simulink model "sim_mdl"  (R2020b)
settings: Solver=FixedStepAuto  StartTime=0.0  StopTime=stoptime  FixedStep=h  MaxStep=1  RelTol=1e-3  AbsTol=1e-6
values from neighbouring files (symbols this model uses):
  ref_select = 1    [Init_general.m]
  strategy_select = 4    [Init_general.m]
undefined symbols (not defined in the file or in its folder): p
settings Model: PauseTimes=3  PacingRate=0.100000  Creator=nobel  LastModifiedBy=natha

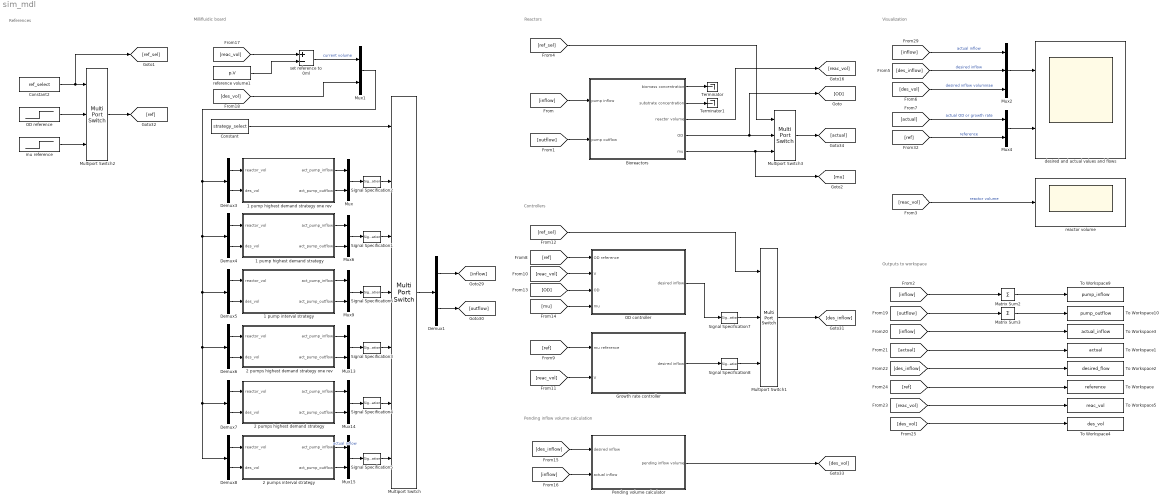
== system sim_mdl ==
  note: Outputs to workspace
  note: Pending inflow volume calculation
  note: Controllers
  note: Millifluidic board
  note: References
  note: Visualization
  note: Reactors
  1 pump highest demand strategy : Stateflow chart  TreatAsAtomicUnit=on  mask{p=p}
      mask prompts: p "Reactor Parameter Struct"
  1 pump highest demand strategy one rev : Stateflow chart  TreatAsAtomicUnit=on  mask{p=p}
      mask prompts: p "Reactor Parameter Struct"
  1 pump interval strategy : Stateflow chart  TreatAsAtomicUnit=on  mask{p=p}
      mask prompts: p "Reactor Parameter Struct"
  2 pumps highest demand strategy : Stateflow chart  TreatAsAtomicUnit=on  mask{p=p}
      mask prompts: p "Reactor Parameter Struct"
  2 pumps highest demand strategy one rev : Stateflow chart  TreatAsAtomicUnit=on  mask{p=p}
      mask prompts: p "Reactor Parameter Struct"
  2 pumps interval strategy : Stateflow chart  TreatAsAtomicUnit=on  mask{p=p}
      mask prompts: p "Reactor Parameter Struct"
  Bioreactors : Subsystem  mask{p=p}
      mask prompts: p "Reactor Parameter Struct"
  Constant : Constant  Value=strategy_select
  Constant2 : Constant  Value=ref_select
  Demux{1,3..8} (7 alike) : Demux  Outputs=2
  Growth rate controller : Subsystem  mask{p=p}
      mask prompts: p "Reactor Parameter Struct"
  Matrix Sum2 : Sum  Inputs=+
  Matrix Sum3 : Sum  Inputs=+
  Multiport Switch : MultiPortSwitch  Inputs=6
  Multiport Switch1 : MultiPortSwitch  Inputs=2
  Multiport Switch2 : MultiPortSwitch  Inputs=2
  Multiport Switch3 : MultiPortSwitch  Inputs=2
  Mux{,1,4,6,9,13..15} (8 alike) : Mux  Inputs=2
  Mux2 : Mux  Inputs=3
  OD controller : Subsystem  mask{p=p}
      mask prompts: p "Reactor Parameter Struct"
  OD reference : Step  Time=p.OD.step_time  Before=p.OD.init_val  After=p.OD.final_val  SampleTime=0  mask{p=p}
      mask prompts: p "Reactor Parameter Struct"
  Pending volume calculator : Subsystem
  Signal Specification{1..6} (6 alike) : SignalSpecification  Dimensions=2*p.num_reac
  Signal Specification7 : SignalSpecification  Dimensions=p.num_reac
  Signal Specification8 : SignalSpecification  Dimensions=p.num_reac
  Terminator : Terminator
  Terminator1 : Terminator
  To Workspace : ToWorkspace  VariableName=reference  SampleTime=-1
  To Workspace1 : ToWorkspace  VariableName=actual  SampleTime=-1
  To Workspace10 : ToWorkspace  VariableName=pump_outflow  SampleTime=-1
      settings: Save2DSignal=2-D array (concatenate along first dimension)
  To Workspace2 : ToWorkspace  VariableName=desired_flow  SampleTime=-1
  To Workspace3 : ToWorkspace  VariableName=actual_inflow  SampleTime=-1
      settings: Save2DSignal=2-D array (concatenate along first dimension)
  To Workspace4 : ToWorkspace  VariableName=des_vol  SampleTime=-1
  To Workspace5 : ToWorkspace  VariableName=reac_vol  SampleTime=-1
  To Workspace9 : ToWorkspace  VariableName=pump_inflow  SampleTime=-1
      settings: Save2DSignal=2-D array (concatenate along first dimension)
  desired and actual values and flows : Scope  NumInputPorts=2
  mu reference : Step  Time=p.growth_rate.step_time  Before=p.growth_rate.init_val  After=p.growth_rate.final_val  SampleTime=0  mask{p=p}
      mask prompts: p "Reactor Parameter Struct"
  reactor volume : Scope
  reference volume1 : Constant  Value=p.V  mask{p=p}
      mask prompts: p "Reactor Parameter Struct"
  set reference to 0ml : Sum  Inputs=+-
  wires:
  Multiport Switch2/1 -> [ref]
  Demux1/2 -> [outflow]
  Demux1/1 -> [inflow]
  [ref] -> Mux4/2  "reference"
  [des_inflow] -> Mux2/2  "desired inflow"
  [des_vol] -> Mux2/3  "desired inflow voluminae"
  Mux4/1 -> desired and actual values and flows/2
  [actual] -> Mux4/1  "actual OD or growth rate"
  [inflow] -> Mux2/1  "actual inflow"
  Mux2/1 -> desired and actual values and flows/1
  [reac_vol] -> reactor volume/1  "reactor volume"
  Mux6/1 -> Signal Specification1/1
  Mux/1 -> Signal Specification2/1
  Demux5/1 -> 1 pump interval strategy/1(reactor_vol)
  Demux4/1 -> 1 pump highest demand strategy/1(reactor_vol)
  1 pump highest demand strategy/2(act_pump_outflow) -> Mux6/2
  Demux3/2 -> 1 pump highest demand strategy one rev/2(des_vol)
  1 pump interval strategy/1(act_pump_inflow) -> Mux9/1
  1 pump highest demand strategy one rev/2(act_pump_outflow) -> Mux/2
  1 pump highest demand strategy one rev/1(act_pump_inflow) -> Mux/1
  1 pump interval strategy/2(act_pump_outflow) -> Mux9/2
  Demux4/2 -> 1 pump highest demand strategy/2(des_vol)
  Demux3/1 -> 1 pump highest demand strategy one rev/1(reactor_vol)
  1 pump highest demand strategy/1(act_pump_inflow) -> Mux6/1
  Demux5/2 -> 1 pump interval strategy/2(des_vol)
  Mux9/1 -> Signal Specification6/1
  Constant/1 -> Multiport Switch/1
  OD reference/1 -> Multiport Switch2/2
  Multiport Switch/1 -> Demux1/1
  Signal Specification6/1 -> Multiport Switch/4
  Signal Specification1/1 -> Multiport Switch/3
  Signal Specification2/1 -> Multiport Switch/2
  Demux7/2 -> 2 pumps highest demand strategy/2(des_vol)
  Demux8/1 -> 2 pumps interval strategy/1(reactor_vol)
  Demux6/2 -> 2 pumps highest demand strategy one rev/2(des_vol)
  Mux14/1 -> Signal Specification4/1
  2 pumps highest demand strategy/1(act_pump_inflow) -> Mux14/1
  2 pumps interval strategy/2(act_pump_outflow) -> Mux15/2
  Mux15/1 -> Signal Specification5/1
  Demux7/1 -> 2 pumps highest demand strategy/1(reactor_vol)
  2 pumps highest demand strategy one rev/1(act_pump_inflow) -> Mux13/1
  2 pumps highest demand strategy/2(act_pump_outflow) -> Mux14/2
  Demux6/1 -> 2 pumps highest demand strategy one rev/1(reactor_vol)
  Demux8/2 -> 2 pumps interval strategy/2(des_vol)
  2 pumps highest demand strategy one rev/2(act_pump_outflow) -> Mux13/2
  2 pumps interval strategy/1(act_pump_inflow) -> Mux15/1  "actual inflow"
  Mux13/1 -> Signal Specification3/1
  Signal Specification5/1 -> Multiport Switch/7
  Signal Specification3/1 -> Multiport Switch/5
  Signal Specification4/1 -> Multiport Switch/6
  [inflow] -> Bioreactors/1(pump inflow)
  [outflow] -> Bioreactors/2(pump outflow)
  Bioreactors/3(reactor volume) -> [reac_vol]
  Bioreactors/4(OD) -> Multiport Switch3/2, [OD]
  Bioreactors/5(mu) -> [mu], Multiport Switch3/3
  Bioreactors/1(biomass concentration) -> Terminator/1
  Bioreactors/2(substrate concentration) -> Terminator1/1
  mu reference/1 -> Multiport Switch2/3
  Constant2/1 -> [ref_sel], Multiport Switch2/1
  Pending volume calculator/1(pending inflow volume) -> [des_vol]
  OD controller/1(desired inflow) -> Signal Specification7/1
  Multiport Switch1/1 -> [des_inflow]
  Growth rate controller/1(desired inflow) -> Signal Specification8/1
  [ref_sel] -> Multiport Switch3/1
  Multiport Switch3/1 -> [actual]
  [ref] -> OD controller/1(OD reference)
  [ref] -> Growth rate controller/1(mu reference)
  [reac_vol] -> OD controller/2(V)
  [reac_vol] -> Growth rate controller/2(V)
  [ref_sel] -> Multiport Switch1/1
  [OD] -> OD controller/3(OD)
  [mu] -> OD controller/4(mu)
  [des_inflow] -> Pending volume calculator/1(desired inflow)
  [inflow] -> Pending volume calculator/2(actual inflow)
  [reac_vol] -> set reference to 0ml/1
  set reference to 0ml/1 -> Mux1/1  "current volume"
  reference volume1/1 -> set reference to 0ml/2
  [des_vol] -> Mux1/2
  Mux1/1 -> Demux3/1, Demux4/1, Demux8/1, Demux7/1, Demux6/1, Demux5/1
  Signal Specification7/1 -> Multiport Switch1/2
  Signal Specification8/1 -> Multiport Switch1/3
  Matrix Sum2/1 -> To Workspace9/1
  [inflow] -> Matrix Sum2/1
  Matrix Sum3/1 -> To Workspace10/1
  [outflow] -> Matrix Sum3/1
  [inflow] -> To Workspace3/1
  [actual] -> To Workspace1/1
  [des_inflow] -> To Workspace2/1
  [ref] -> To Workspace/1
  [reac_vol] -> To Workspace5/1
  [des_vol] -> To Workspace4/1

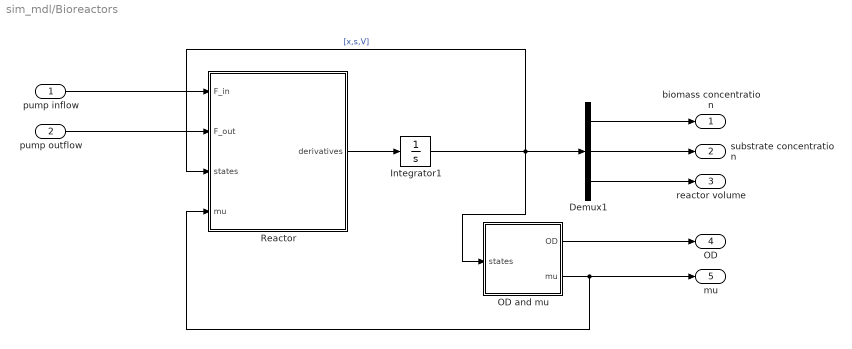
== system sim_mdl/Bioreactors ==
  pump inflow : Inport
  pump outflow : Inport  Port=2
  Demux1 : Demux  Outputs=3
  Integrator1 : Integrator  InitialCondition=[p.init_x; p.init_s; p.init_v];
  OD and mu : MATLAB Function  TreatAsAtomicUnit=on
  Reactor : MATLAB Function  TreatAsAtomicUnit=on
  biomass concentration : Outport
  substrate concentration : Outport  Port=2
  reactor volume : Outport  Port=3
  OD : Outport  Port=4
  mu : Outport  Port=5
  wires:
  pump inflow/1 -> Reactor/1(F_in)
  Demux1/3 -> reactor volume/1
  pump outflow/1 -> Reactor/2(F_out)
  Reactor/1(derivatives) -> Integrator1/1
  OD and mu/2(mu) -> Reactor/4(mu), mu/1
  OD and mu/1(OD) -> OD/1
  Demux1/2 -> substrate concentration/1
  Demux1/1 -> biomass concentration/1
  Integrator1/1 -> Reactor/3(states), Demux1/1, OD and mu/1(states)  "[x,s,V]"

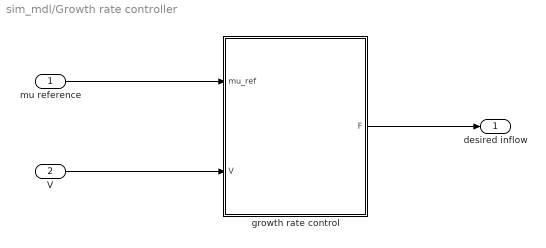
== system sim_mdl/Growth rate controller ==
  mu reference : Inport
  V : Inport  Port=2
  growth rate control : MATLAB Function  TreatAsAtomicUnit=on
  desired inflow : Outport
  wires:
  growth rate control/1(F) -> desired inflow/1
  V/1 -> growth rate control/2(V)
  mu reference/1 -> growth rate control/1(mu_ref)

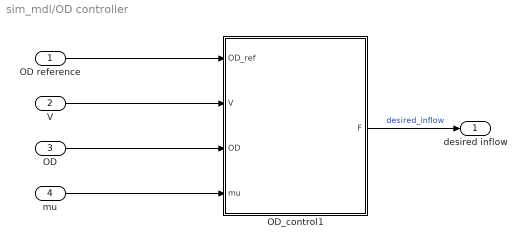
== system sim_mdl/OD controller ==
  OD reference : Inport
  V : Inport  Port=2
  OD : Inport  Port=3
  mu : Inport  Port=4
  OD_control1 : MATLAB Function  TreatAsAtomicUnit=on
  desired inflow : Outport
  wires:
  OD reference/1 -> OD_control1/1(OD_ref)
  mu/1 -> OD_control1/4(mu)
  V/1 -> OD_control1/2(V)
  OD/1 -> OD_control1/3(OD)
  OD_control1/1(F) -> desired inflow/1  "desired_inflow"

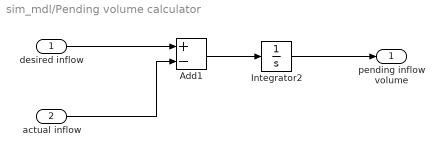
== system sim_mdl/Pending volume calculator ==
  desired inflow : Inport
  actual inflow : Inport  Port=2
  Add1 : Sum  Inputs=+-
  Integrator2 : Integrator  InitialCondition=zeros(p.num_reac,1)
  pending inflow volume : Outport
  wires:
  Add1/1 -> Integrator2/1
  desired inflow/1 -> Add1/1
  actual inflow/1 -> Add1/2
  Integrator2/1 -> pending inflow volume/1

== stateflow chart sim_mdl/1 pump interval strategy ==
  state procedures [parallel]
    settings: executionOrder=3
    state normal
    state sampling
      entry: sampling_req=true;
    (default) -> normal
    normal -> sampling : after(p.sampling_int, sec)
    sampling -> normal : sampling_done
  state counter [parallel]
    settings: executionOrder=1
    state init_counter
      entry: reac_ind = 1;
    state increase_counter
      entry: reac_ind = reac_ind+1;
    state cycle_over
    (default) -> init_counter : % loop_counter
    increase_counter -> (junction 211) : after(p.interval/p.num_reac,sec)
    (junction 211) -> cycle_over [order 2]
    (junction 211) -> increase_counter [order 1] : [reac_ind<p.num_reac]
    init_counter -> increase_counter : after(p.interval/p.num_reac,sec)
    cycle_over -> init_counter : next_cycle
  state feeding_wasting_sampling [parallel]
    settings: executionOrder=2
    state inflow
      state inflow_act
        entry: vol_pump_in=floor(des_vol(reac_ind)/...
        p.pump_res)*p.pump_res;
        act_pump_inflow(reac_ind)=p.max_pump_flow;
      state inflow_inact
        entry: act_pump_inflow(:)=0;
      inflow_act -> inflow_inact [order 3] : [vol_pump_in<=0]
      inflow_act -> inflow_inact [order 1] : after(vol_pump_in/p.max_pump_flow,sec)
      inflow_inact -> inflow_act [order 1] : enter(counter.increase_counter)
      inflow_act -> inflow_inact [order 2] : after(p.interval/p.num_reac-1e-3,sec)
    state outflow_waste
      state outflow_act
        entry: vol_pump_out=reactor_vol(reac_ind);
        act_pump_outflow(reac_ind)=p.max_pump_flow;
      state outflow_inact
        entry: act_pump_outflow(:)=0;
      feeding_wasting_sampling.outflow_waste.outflow_act -> feeding_wasting_sampling.outflow_waste.outflow_inact [order 3] : [vol_pump_out<=0]
      feeding_wasting_sampling.outflow_waste.outflow_act -> feeding_wasting_sampling.outflow_waste.outflow_inact [order 1] : after(vol_pump_out/p.max_pump_flow,sec)
      feeding_wasting_sampling.outflow_waste.outflow_inact -> feeding_wasting_sampling.outflow_waste.outflow_act [order 1] : enter(counter.increase_counter)
      feeding_wasting_sampling.outflow_waste.outflow_act -> feeding_wasting_sampling.outflow_waste.outflow_inact [order 2] : after(p.interval/p.num_reac-1e-3,sec)
    state cleaning_procedure
    state outflow_sampling
      state outflow_act
        entry: vol_pump_out=p.pump_res;
        act_pump_outflow(reac_ind)=p.max_pump_flow;
      state outflow_inact
        entry: act_pump_outflow(:)=0;
      feeding_wasting_sampling.outflow_sampling.outflow_act -> feeding_wasting_sampling.outflow_sampling.outflow_inact : after(vol_pump_out/p.max_pump_flow,sec)
      feeding_wasting_sampling.outflow_sampling.outflow_inact -> feeding_wasting_sampling.outflow_sampling.outflow_act [order 1] : enter(counter.increase_counter)
    (default) -> inflow_act
    (junction 263) -> inflow_act [order 2] : [in(procedures.normal)]{send(next_cycle,counter)}
    inflow_inact -> feeding_wasting_sampling.outflow_waste.outflow_act [order 2] : enter(counter.cycle_over) {send(next_cycle,counter)}
    feeding_wasting_sampling.outflow_waste.outflow_inact -> inflow_act [order 3] : [enter(counter.cycle_over) && in(procedures.normal)]{send(next_cycle,counter)}
    feeding_wasting_sampling.outflow_waste.outflow_inact -> cleaning_procedure [order 2] : [enter(counter.cycle_over)]
    feeding_wasting_sampling.outflow_sampling.outflow_inact -> cleaning_procedure [order 2] : [enter(counter.cycle_over)]{send(sampling_done, procedures)}
    cleaning_procedure -> (junction 263) : after(p.clean_time,sec)
    (junction 263) -> feeding_wasting_sampling.outflow_sampling.outflow_act [order 1] : [in(procedures.sampling)] {send(next_cycle,counter)}
  data: act_pump_inflow output size=p.num_reac =zeros(p.num_reac,1); reactor_vol input size=p.num_reac; des_vol input size=p.num_reac; vol_pump_in local; act_pump_outflow output size=p.num_reac =zeros(p.num_reac,1); vol_pump_out local; reac_ind local; sampling_req local; p parameter
  events: sampling_done local FUNCTION_CALL_EVENT; next_cycle local FUNCTION_CALL_EVENT

== stateflow chart sim_mdl/1 pump highest demand strategy ==
  state procedures [parallel]
    settings: executionOrder=2
    state normal
    state sampling
      entry: sampling_req=true;
    (default) -> normal
    normal -> sampling : after(p.sampling_int, sec)
    sampling -> normal : sampling_done
  state feeding_wasting_sampling [parallel]
    settings: executionOrder=1
    state feeding
      state inflow
        state inflow_act
          entry: act_pump_inflow(reac_ind)=p.max_pump_flow;
          vol_pump_in = floor(vol_pump_in/p.pump_res)*p.pump_res;
        state inflow_inact
          entry: act_pump_inflow(:)=0;
          [vol_pump_in, reac_ind] = max(des_vol);
          during: [vol_pump_in, reac_ind] = max(des_vol);
        inflow_act -> inflow_inact [order 1] : after(vol_pump_in/p.max_pump_flow,sec)
        inflow_act -> inflow_inact [order 2] : [vol_pump_in<=0]
        inflow_inact -> inflow_act [order 2] : [vol_pump_in>=p.pump_res]
    state outflow_waste
      state outflow_act
        entry: act_pump_outflow(reac_ind)=...
        p.max_pump_flow;
        vol_pump_out = reactor_vol(reac_ind);
        % vol_pump_out = floor(reactor_vol(reac_ind)/...
        % p.pump_res)*p.pump_res;
      state outflow_inact
        entry: act_pump_outflow(:)=0;
      feeding_wasting_sampling.outflow_waste.outflow_act -> feeding_wasting_sampling.outflow_waste.outflow_inact [order 1] : [vol_pump_out<=0]
      feeding_wasting_sampling.outflow_waste.outflow_act -> feeding_wasting_sampling.outflow_waste.outflow_inact [order 2] : after(vol_pump_out/p.max_pump_flow,sec)
      feeding_wasting_sampling.outflow_waste.outflow_inact -> feeding_wasting_sampling.outflow_waste.outflow_act [order 2] : {reac_ind = reac_ind+1;}
    state cleaning_procedure
    state outflow_sampling
      state outflow_act
        entry: vol_pump_out=p.pump_res;
        act_pump_outflow(reac_ind)=p.max_pump_flow;
      state outflow_inact
        entry: act_pump_outflow(:)=0;
      feeding_wasting_sampling.outflow_sampling.outflow_act -> feeding_wasting_sampling.outflow_sampling.outflow_inact : after(vol_pump_out/p.max_pump_flow,sec)
      feeding_wasting_sampling.outflow_sampling.outflow_inact -> feeding_wasting_sampling.outflow_sampling.outflow_act [order 2] : {reac_ind=reac_ind+1;}
    (junction 263) -> inflow_inact [order 2] : [in(procedures.normal)]
    inflow_inact -> feeding_wasting_sampling.outflow_waste.outflow_act [order 1] : [sum(reactor_vol>p.waste_threshold)>0]{reac_ind=1;}
    cleaning_procedure -> (junction 263) : after(p.clean_time,sec)
    (junction 263) -> feeding_wasting_sampling.outflow_sampling.outflow_act [order 1] : [in(procedures.sampling)]{reac_ind=1;}
    feeding_wasting_sampling.outflow_sampling.outflow_inact -> cleaning_procedure [order 1] : [reac_ind==p.num_reac]{send(sampling_done,procedures)}
    feeding_wasting_sampling.outflow_waste.outflow_inact -> cleaning_procedure [order 1] : [reac_ind == p.num_reac]
  (default) -> inflow_inact
  data: act_pump_inflow output size=p.num_reac =zeros(p.num_reac,1); reactor_vol input size=p.num_reac; des_vol input size=p.num_reac; vol_pump_in local; act_pump_outflow output size=p.num_reac =zeros(p.num_reac,1); vol_pump_out local; sampling_req local; p parameter; reac_ind local =1
  events: sampling_done local FUNCTION_CALL_EVENT

== stateflow chart sim_mdl/1 pump highest demand strategy one rev ==
  state procedures [parallel]
    settings: executionOrder=2
    state normal
    state sampling
      entry: sampling_req=true;
    (default) -> normal
    normal -> sampling : after(p.sampling_int, sec)
    sampling -> normal : sampling_done
  state feeding_wasting_sampling [parallel]
    settings: executionOrder=1
    state feeding
      state inflow
        state inflow_act
          entry: act_pump_inflow(reac_ind)=p.max_pump_flow;
        state inflow_inact
          entry: act_pump_inflow(:)=0;
          [vol_pump_in, reac_ind] = max(des_vol);
          during: [vol_pump_in, reac_ind] = max(des_vol);
        inflow_act -> inflow_inact [order 1] : after(p.pump_res/p.max_pump_flow,sec)
        inflow_act -> inflow_inact [order 2] : [vol_pump_in<=0]
        inflow_inact -> inflow_act [order 2] : [vol_pump_in>=p.pump_res]
    state outflow_waste
      state outflow_act
        entry: act_pump_outflow(reac_ind)=...
        p.max_pump_flow;
        vol_pump_out = reactor_vol(reac_ind);
        % vol_pump_out = floor(reactor_vol(reac_ind)/...
        % p.pump_res)*p.pump_res;
      state outflow_inact
        entry: act_pump_outflow(:)=0;
      feeding_wasting_sampling.outflow_waste.outflow_act -> feeding_wasting_sampling.outflow_waste.outflow_inact [order 1] : [vol_pump_out<=0]
      feeding_wasting_sampling.outflow_waste.outflow_act -> feeding_wasting_sampling.outflow_waste.outflow_inact [order 2] : after(vol_pump_out/p.max_pump_flow,sec)
      feeding_wasting_sampling.outflow_waste.outflow_inact -> feeding_wasting_sampling.outflow_waste.outflow_act [order 2] : {reac_ind = reac_ind+1;}
    state cleaning_procedure
    state outflow_sampling
      state outflow_act
        entry: vol_pump_out=p.pump_res;
        act_pump_outflow(reac_ind)=p.max_pump_flow;
      state outflow_inact
        entry: act_pump_outflow(:)=0;
      feeding_wasting_sampling.outflow_sampling.outflow_act -> feeding_wasting_sampling.outflow_sampling.outflow_inact : after(vol_pump_out/p.max_pump_flow,sec)
      feeding_wasting_sampling.outflow_sampling.outflow_inact -> feeding_wasting_sampling.outflow_sampling.outflow_act [order 2] : {reac_ind=reac_ind+1;}
    (junction 263) -> inflow_inact [order 2] : [in(procedures.normal)]
    inflow_inact -> feeding_wasting_sampling.outflow_waste.outflow_act [order 1] : [sum(reactor_vol>p.waste_threshold)>0]{reac_ind=1;}
    cleaning_procedure -> (junction 263) : after(p.clean_time,sec)
    (junction 263) -> feeding_wasting_sampling.outflow_sampling.outflow_act [order 1] : [in(procedures.sampling)]{reac_ind=1;}
    feeding_wasting_sampling.outflow_sampling.outflow_inact -> cleaning_procedure [order 1] : [reac_ind==p.num_reac]{send(sampling_done,procedures)}
    feeding_wasting_sampling.outflow_waste.outflow_inact -> cleaning_procedure [order 1] : [reac_ind == p.num_reac]
  (default) -> inflow_inact
  data: act_pump_inflow output size=p.num_reac =zeros(p.num_reac,1); reactor_vol input size=p.num_reac; des_vol input size=p.num_reac; vol_pump_in local; act_pump_outflow output size=p.num_reac =zeros(p.num_reac,1); vol_pump_out local; sampling_req local; p parameter; reac_ind local =1
  events: sampling_done local FUNCTION_CALL_EVENT

== stateflow chart sim_mdl/2 pumps highest demand strategy one rev ==
  state procedures [parallel]
    settings: executionOrder=1
    state normal
    state sampling
      entry: sampling_req=true;
    (default) -> normal
    normal -> sampling : after(p.sampling_int, sec)
    sampling -> normal : sampling_done
  state feeding [parallel]
    settings: executionOrder=2
    state inflow
      state inflow_act
        entry: act_pump_inflow(reac_ind_inflow)=...
        p.max_pump_flow;
      state inflow_inact
        entry: act_pump_inflow(:)=0;
        [vol_pump_in, reac_ind_inflow] = max(des_vol);
        during: [vol_pump_in, reac_ind_inflow] = max(des_vol);
      inflow_act -> inflow_inact [order 1] : after(p.pump_res/p.max_pump_flow,sec)
      inflow_act -> inflow_inact [order 2] : [vol_pump_in<=0]
      inflow_inact -> inflow_act : [vol_pump_in>=p.pump_res]
    (default) -> inflow_inact
  state wasting_sampling [parallel]
    settings: executionOrder=3
    state outflow_waste
      state outflow_act
        entry: act_pump_outflow(reac_ind_outflow)=...
        p.max_pump_flow;
      state outflow_inact
        entry: act_pump_outflow(:)=0;
        [vol_pump_out, reac_ind_outflow] = max(reactor_vol);
        during: [vol_pump_out, reac_ind_outflow] = ...
        max(reactor_vol);
      wasting_sampling.outflow_waste.outflow_act -> wasting_sampling.outflow_waste.outflow_inact [order 1] : [vol_pump_out<=0]
      wasting_sampling.outflow_waste.outflow_act -> wasting_sampling.outflow_waste.outflow_inact [order 2] : after(vol_pump_out/p.max_pump_flow,sec)
      wasting_sampling.outflow_waste.outflow_inact -> wasting_sampling.outflow_waste.outflow_act [order 2] : [vol_pump_out>=p.pump_res]
    state cleaning_procedure
    state outflow_sampling
      state outflow_act
        entry: vol_pump_out=p.pump_res;
        act_pump_outflow(reac_ind_outflow)=p.max_pump_flow;
      state outflow_inact
        entry: act_pump_outflow(:)=0;
      wasting_sampling.outflow_sampling.outflow_act -> wasting_sampling.outflow_sampling.outflow_inact : after(vol_pump_out/p.max_pump_flow,sec)
      wasting_sampling.outflow_sampling.outflow_inact -> wasting_sampling.outflow_sampling.outflow_act [order 2] : {reac_ind_outflow=reac_ind_outflow+1;}
    (default) -> wasting_sampling.outflow_waste.outflow_inact
    wasting_sampling.outflow_waste.outflow_inact -> cleaning_procedure [order 1] : [in(procedures.sampling)]
    wasting_sampling.outflow_sampling.outflow_inact -> wasting_sampling.outflow_waste.outflow_inact [order 1] : [reac_ind_outflow==p.num_reac]{send(sampling_done,procedures)}
    cleaning_procedure -> (junction 263) : after(p.clean_time,sec)
    (junction 263) -> wasting_sampling.outflow_sampling.outflow_act : {reac_ind_outflow=1;}
  data: act_pump_inflow output size=p.num_reac =zeros(p.num_reac,1); reactor_vol input size=p.num_reac; des_vol input size=p.num_reac; vol_pump_in local; act_pump_outflow output size=p.num_reac =zeros(p.num_reac,1); vol_pump_out local; reac_ind_inflow local =1; sampling_req local; p parameter; reac_ind_outflow local =1
  events: sampling_done local FUNCTION_CALL_EVENT

== stateflow chart sim_mdl/2 pumps highest demand strategy ==
  state procedures [parallel]
    settings: executionOrder=1
    state normal
    state sampling
      entry: sampling_req=true;
    (default) -> normal
    normal -> sampling : after(p.sampling_int, sec)
    sampling -> normal : sampling_done
  state feeding [parallel]
    settings: executionOrder=2
    state inflow
      state inflow_act
        entry: act_pump_inflow(reac_ind_inflow)=...
        p.max_pump_flow;
        vol_pump_in = floor(vol_pump_out/p.pump_res)...
        *p.pump_res;
      state inflow_inact
        entry: act_pump_inflow(:)=0;
        [vol_pump_in, reac_ind_inflow] = max(des_vol);
        during: [vol_pump_in, reac_ind_inflow] = max(des_vol);
      inflow_act -> inflow_inact [order 1] : after(vol_pump_in/p.max_pump_flow,sec)
      inflow_act -> inflow_inact [order 2] : [vol_pump_in<=0]
      inflow_inact -> inflow_act : [vol_pump_in>=p.pump_res]
    (default) -> inflow_inact
  state wasting_sampling [parallel]
    settings: executionOrder=3
    state outflow_waste
      state outflow_act
        entry: act_pump_outflow(reac_ind_outflow)=...
        p.max_pump_flow;
        % vol_pump_out = floor(vol_pump_out/p.pump_res)...
        % *p.pump_res;
      state outflow_inact
        entry: act_pump_outflow(:)=0;
        [vol_pump_out, reac_ind_outflow] = max(reactor_vol);
        during: [vol_pump_out, reac_ind_outflow] = ...
        max(reactor_vol);
      wasting_sampling.outflow_waste.outflow_act -> wasting_sampling.outflow_waste.outflow_inact [order 1] : [vol_pump_out<=0]
      wasting_sampling.outflow_waste.outflow_act -> wasting_sampling.outflow_waste.outflow_inact [order 2] : after(vol_pump_out/p.max_pump_flow,sec)
      wasting_sampling.outflow_waste.outflow_inact -> wasting_sampling.outflow_waste.outflow_act [order 2] : [vol_pump_out>=p.pump_res]
    state cleaning_procedure
    state outflow_sampling
      state outflow_act
        entry: vol_pump_out=p.pump_res;
        act_pump_outflow(reac_ind_outflow)=p.max_pump_flow;
      state outflow_inact
        entry: act_pump_outflow(:)=0;
      wasting_sampling.outflow_sampling.outflow_act -> wasting_sampling.outflow_sampling.outflow_inact : after(vol_pump_out/p.max_pump_flow,sec)
      wasting_sampling.outflow_sampling.outflow_inact -> wasting_sampling.outflow_sampling.outflow_act [order 2] : {reac_ind_outflow=reac_ind_outflow+1;}
    (default) -> wasting_sampling.outflow_waste.outflow_inact
    wasting_sampling.outflow_waste.outflow_inact -> cleaning_procedure [order 1] : [in(procedures.sampling)]
    wasting_sampling.outflow_sampling.outflow_inact -> wasting_sampling.outflow_waste.outflow_inact [order 1] : [reac_ind_outflow==p.num_reac]{send(sampling_done,procedures)}
    cleaning_procedure -> (junction 263) : after(p.clean_time,sec)
    (junction 263) -> wasting_sampling.outflow_sampling.outflow_act : {reac_ind_outflow=1;}
  data: act_pump_inflow output size=p.num_reac =zeros(p.num_reac,1); reactor_vol input size=p.num_reac; des_vol input size=p.num_reac; vol_pump_in local; act_pump_outflow output size=p.num_reac =zeros(p.num_reac,1); vol_pump_out local; reac_ind_inflow local =1; sampling_req local; p parameter; reac_ind_outflow local =1
  events: sampling_done local FUNCTION_CALL_EVENT

== stateflow chart sim_mdl/2 pumps interval strategy ==
  state counter_inflow [parallel]
    settings: executionOrder=1
    state init_counter
      entry: reac_ind_inflow = 1;
    state increase_counter
      entry: reac_ind_inflow = reac_ind_inflow+1;
    state cycle_over
    (default) -> counter_inflow.init_counter : % loop_counter
    (junction 211) -> counter_inflow.cycle_over [order 2]
    (junction 211) -> counter_inflow.increase_counter [order 1] : [reac_ind_inflow<p.num_reac]
    counter_inflow.increase_counter -> (junction 211) : after(p.interval/p.num_reac,sec)
    counter_inflow.init_counter -> counter_inflow.increase_counter : after(p.interval/p.num_reac,sec)
    counter_inflow.cycle_over -> counter_inflow.init_counter
  state counter_outflow [parallel]
    settings: executionOrder=4
    state init_counter
      entry: reac_ind_outflow = 1;
    state increase_counter
      entry: reac_ind_outflow = reac_ind_outflow+1;
    state cycle_over
    (default) -> counter_outflow.init_counter : % loop_counter
    (junction 274) -> counter_outflow.cycle_over [order 2]
    (junction 274) -> counter_outflow.increase_counter [order 1] : [reac_ind_outflow<p.num_reac]
    counter_outflow.increase_counter -> (junction 274) : after(p.interval/p.num_reac,sec)
    counter_outflow.init_counter -> counter_outflow.increase_counter : after(p.interval/p.num_reac,sec)
    counter_outflow.cycle_over -> counter_outflow.init_counter : next_cycle
  state procedures [parallel]
    settings: executionOrder=3
    state normal
    state sampling
      entry: sampling_req=true;
    (default) -> normal
    normal -> sampling : after(p.sampling_int, sec)
    sampling -> normal : sampling_done
  state feeding [parallel]
    settings: executionOrder=5
    state inflow
      state inflow_act
        entry: vol_pump_in=floor(des_vol(reac_ind_inflow)/...
        p.pump_res)*p.pump_res;
        act_pump_inflow(reac_ind_inflow)=p.max_pump_flow;
      state inflow_inact
        entry: act_pump_inflow(:)=0;
      inflow_act -> inflow_inact [order 3] : [vol_pump_in<=0]
      inflow_act -> inflow_inact [order 1] : after(vol_pump_in/p.max_pump_flow,sec)
      inflow_inact -> inflow_act [order 1] : enter(counter_inflow.increase_counter)
      inflow_inact -> inflow_act [order 2] : enter(counter_inflow.init_counter)
      inflow_act -> inflow_inact [order 2] : after(p.interval/p.num_reac-1e-3,sec)
    (default) -> inflow_act
  state wasting_sampling [parallel]
    settings: executionOrder=2
    state outflow_waste
      state outflow_act
        entry:vol_pump_out = reactor_vol(reac_ind_outflow);
        %vol_pump_out=...
        %  floor(reactor_vol(reac_ind_outflow)/...
        %  p.pump_res)*p.pump_res;
        act_pump_outflow(reac_ind_outflow)=p.max_pump_flow;
      state outflow_inact
        entry: act_pump_outflow(:)=0;
      wasting_sampling.outflow_waste.outflow_inact -> wasting_sampling.outflow_waste.outflow_act [order 1] : [enter(counter_outflow.cycle_over) && in(procedures.normal)]{send(next_cycle,counter_outflow)}
      wasting_sampling.outflow_waste.outflow_act -> wasting_sampling.outflow_waste.outflow_inact [order 1] : [vol_pump_out<=0]
      wasting_sampling.outflow_waste.outflow_act -> wasting_sampling.outflow_waste.outflow_inact [order 2] : after(vol_pump_out/p.max_pump_flow,sec)
      wasting_sampling.outflow_waste.outflow_inact -> wasting_sampling.outflow_waste.outflow_act [order 2] : enter(counter_outflow.increase_counter)
      wasting_sampling.outflow_waste.outflow_act -> wasting_sampling.outflow_waste.outflow_inact [order 3] : after(p.interval/p.num_reac-1e-3,sec)
    state cleaning_procedure
    state outflow_sampling
      state outflow_act
        entry: vol_pump_out=p.pump_res;
        act_pump_outflow(reac_ind_outflow)=...
        p.max_pump_flow;
      state outflow_inact
        entry: act_pump_outflow(:)=0;
      wasting_sampling.outflow_sampling.outflow_act -> wasting_sampling.outflow_sampling.outflow_inact : after(vol_pump_out/p.max_pump_flow,sec)
      wasting_sampling.outflow_sampling.outflow_inact -> wasting_sampling.outflow_sampling.outflow_act [order 1] : enter(counter_outflow.increase_counter)
    (default) -> wasting_sampling.outflow_waste.outflow_act
    wasting_sampling.outflow_waste.outflow_inact -> cleaning_procedure [order 3] : [enter(counter_outflow.cycle_over) && in(procedures.sampling)]
    wasting_sampling.outflow_sampling.outflow_inact -> wasting_sampling.outflow_waste.outflow_act [order 2] : [enter(counter_outflow.cycle_over)]{send(sampling_done, procedures);send(next_cycle, counter_outflow)}
    cleaning_procedure -> (junction 263) : after(p.clean_time,sec)
    (junction 263) -> wasting_sampling.outflow_sampling.outflow_act : {send(next_cycle,counter_outflow)}
  data: act_pump_inflow output size=p.num_reac =zeros(p.num_reac,1); reactor_vol input size=p.num_reac; des_vol input size=p.num_reac; vol_pump_in local; act_pump_outflow output size=p.num_reac =zeros(p.num_reac,1); vol_pump_out local; reac_ind_inflow local =1; sampling_req local; p parameter; reac_ind_outflow local =1
  events: sampling_done local FUNCTION_CALL_EVENT; next_cycle local FUNCTION_CALL_EVENT

== matlab function sim_mdl/OD controller/OD_control1 ==
  data: OD_ref input; V input; F output; OD input; mu input
function F = fcn(OD_ref,V,OD,mu)

F = OD.*mu./OD_ref.*V;

== matlab function sim_mdl/Bioreactors/Reactor ==
  data: F_in input; derivatives output size=3*p.num_reac; F_out input; states input; mu input; p parameter
function derivatives   = fcn(F_in,F_out,states, mu, p)

x=states(1:p.num_reac);
s=states(p.num_reac+(1:p.num_reac));
V=states(2*p.num_reac+(1:p.num_reac));

D = F_in./V;

%dx    (Concentration of biomass in the biorreactor)
dx= mu.*x - D.*x;

%ds    (Concentration of substrate in the biorreactor)
ds= -p.y.*mu.*x + D.*(p.s_f - s);

%dV    (Volume of liquid inside the biorreactor)
dV= F_in - F_out;


derivatives = [dx; ds; dV];

== matlab function sim_mdl/Bioreactors/OD and mu ==
  data: states input; OD output; mu output; p parameter
function [OD,mu] = fcn(states, p)

x=states(1:p.num_reac);
s=states(p.num_reac+(1:p.num_reac));
V=states(2*p.num_reac+(1:p.num_reac));

OD=x./p.m_p./p.nOD;
mu = p.mu_max.*s./(p.K_s+s);

== matlab function sim_mdl/Growth rate controller/growth rate control ==
  data: mu_ref input; V input; F output
function F = fcn(mu_ref,V)

F = mu_ref.*V;
